simulink library "SensLib"  (R2016b)
settings: Solver=ode45  StartTime=0.0  StopTime=10.0  RelTol=1e-3  EnableMultiTasking=on
undefined symbols (not defined in the file or in its folder): AC, sens
libraries: SensLib x47, OpenFlightUtilLib x8, simulink x2
settings Model: Creator=University of Minnesota  LastModifiedBy=rega0051
settings DataIOCC: LimitDataPoints=on  SaveFormat=Array  SignalLoggingSaveFormat=ModelDataLogs
settings OptimizationCC: ExpressionDepthLimit=2147483647  LifeSpan=inf  SimCompilerOptimization=on
settings DebuggingCC: UnderspecifiedInitializationDetection=Classic  MergeDetectMultiDrivingBlocksExec=none  SolverPrmCheckMsg=warning  FcnCallInpInsideContextMsg=warning  StateNameClashWarn=warning  StrictBusMsg=Warning  SFUnexpectedBacktrackingDiag=warning  SFNoUnconditionalDefaultTransitionDiag=warning  SFExecutionAtInitializationDiag=none
settings HardwareCC: ProdBitPerPointer=32  ProdBitPerSizeT=32  ProdBitPerPtrDiffT=32  ProdLargestAtomicFloat=None  ProdIntDivRoundTo=Undefined  ProdEndianess=Unspecified  ProdWordSize=32  ProdHWDeviceType=32-bit Generic
settings ModelReferenceCC: PropagateSignalLabelsOutOfModel=off
settings GRTTargetCC: TargetLangStandard=C89/C90 (ANSI)  GeneratePreprocessorConditionals=Disable all  CombineOutputUpdateFcns=off  GRTInterface=on
settings ConfigComp: CovMetricSettings=dw  CovHtmlReporting=on  CovSaveCumulativeToWorkspaceVar=on  CovSaveSingleToWorkspaceVar=on  CovExternalEMLEnable=off

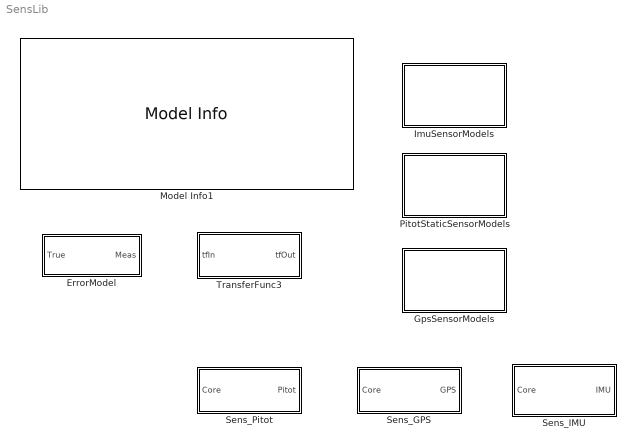
== system SensLib ==
  ErrorModel : Subsystem  mask(Sensor Error Model - Scale, Bias, Noise){enable=sens.errEnable, scf=sens.velScf, bias=sens.velBias, sigma=sens.velSigma, seed=sens.velSeed, timestep=sens.timeSample_s}
      mask prompts: enable "Enable (on/off):"; scf "Scale Factor:"; sigma "Noise Sigma:"; seed "Noise Seed:"; timestep "Time Step (s):"
      mask help:
      | Apply a scale factor, add a bias and noise to a signal.
      |
      | - Enable (on/off): 1 = error on, 0 = error off.
      | - 'Scale Factor' : Scale factor applied to original signal (applied as a matrix multiplication).
      | - 'Bias'  : Constant offset bias (vectorized).
      | - 'Sigma' : Standard deviation of noise (vectorized).
      | - 'Noise Seed'  : Random number seed (vectorized).
      | - 'Time Step (s)': Time step for the noise generation.
      mask Display: disp('bias/scf/noise')
  GpsSensorModels : Subsystem
  ImuSensorModels : Subsystem
  Model Info1 : simulink/Model-Wide Utilities/Model Info  Frame=on  DisplayStringWithTags=|  HorizontalTextAlignment=Left  LeftAlignmentValue=0.02  SourceBlockDiagram=SensLib  TagMaxNumber=20
      | MODEL INFORMATION
      | Sensors Library (%<ModelName>)
      | 
      | University of Minnesota
      | Aerospace Engineering and Mechanics
      | Copyright 2017 Regents of the University of Minnesota. All rights reserved.
      | 
      | == Update Info ==
      | Last modified by %<LastModifiedBy> on %<LastModificationDate>
  PitotStaticSensorModels : Subsystem
  Sens_GPS : Subsystem  TreatAsAtomicUnit=on  VariantControl=Variant1  mask{sens=AC.Sens.GPS}
      mask prompts: sens "GPS Parameter Structure:"
  Sens_IMU : Subsystem  TreatAsAtomicUnit=on  VariantControl=VarImu_LocTransErr  mask{sens=AC.Sens.IMU}
      mask prompts: sens "IMU Parameter Structure:"
  Sens_Pitot : Subsystem  TreatAsAtomicUnit=on  VariantControl=VarAirData_LocTransErr  mask{sens=AC.Sens.Pitot}
      mask prompts: sens "AirData Parameter Structure:"
  TransferFunc3 : Subsystem  mask(Transfer Function (3)){tf_num=sens.gyroTF_num, tf_den=sens.gyroTF_den}
      mask prompts: tf_num "Transfer Function Numerator:"; tf_den "Transfer Function Denominator:"
      mask help: Applies a Transfer Function to a vector signal of length 3. The same transfer function is applied to each signal in the vector.
      settings: AttributesFormatString=%<tf_num> / %<tf_den>

== system SensLib/ErrorModel ==
  True : Inport
  Add1 : Sum  Inputs=+++
  Band-Limited White Noise : simulink/Sources/Band-Limited White Noise  Cov=sigma  Ts=timestep  seed=seed
  Gain : Gain  Gain=scf  Multiplication=Matrix(K*u)
  Gear1 : Constant  Value=bias
  Gear2 : Constant  Value=enable
  Reshape : Reshape  OutputDimensionality=Column vector (2-D)
  Switch : Switch  Criteria=u2 > Threshold
  Meas : Outport
  wires:
  Reshape/1 -> Gain/1
  Band-Limited White Noise/1 -> Add1/3
  Gear1/1 -> Add1/2
  Add1/1 -> Switch/1
  True/1 -> Switch/3, Reshape/1
  Gain/1 -> Add1/1
  Switch/1 -> Meas/1
  Gear2/1 -> Switch/2

== system SensLib/GpsSensorModels ==
  GPS_Err : Subsystem  TreatAsAtomicUnit=on  VariantControl=Variant1
  GPS_LocErr : Subsystem  TreatAsAtomicUnit=on  VariantControl=Variant1
  GPS_LocTransErr : Subsystem  TreatAsAtomicUnit=on  VariantControl=Variant1
  GPS_Pass : Subsystem  TreatAsAtomicUnit=on  VariantControl=Variant1
  Sens_GPS : Subsystem  BlockChoice=GPS_LocErr  mask{sens=AC.Sens.GPS}
      mask prompts: sens "GPS Parameter Structure:"
      settings: TemplateBlock=self  MemberBlocks=GPS_Err,GPS_LocErr,GPS_LocTransErr,GPS_Pass
      settings: AttributesFormatString=|
      | %<BlockChoice>
      | Param Struct: %<sens>

== system SensLib/ImuSensorModels ==
  Body2IMU : Subsystem
  IMU_Err : Subsystem  TreatAsAtomicUnit=on  VariantControl=VarImu_Err
  IMU_LocErr : Subsystem  TreatAsAtomicUnit=on  VariantControl=VarImu_LocErr
  IMU_LocTransErr : Subsystem  TreatAsAtomicUnit=on  VariantControl=VarImu_LocTransErr
  IMU_Pass : Subsystem  TreatAsAtomicUnit=on  VariantControl=VarIMU_Pass
  Sens_IMU : Subsystem  BlockChoice=IMU_LocErr  mask{sens=AC.Sens.IMU}
      mask prompts: sens "Imu Param Struct:"
      settings: TemplateBlock=self  MemberBlocks=IMU_Err,IMU_LocErr,IMU_LocTransErr,IMU_Pass
      settings: AttributesFormatString=|
      | %<BlockChoice>
      | Param Struct: %<sens>

== system SensLib/PitotStaticSensorModels ==
  Body2PitotStatic : Subsystem
  Pitot_Err : Subsystem  TreatAsAtomicUnit=on  VariantControl=Variant1
  Pitot_LocErr : Subsystem  TreatAsAtomicUnit=on  VariantControl=VarAirData_LocErr
  Pitot_LocTransErr : Subsystem  TreatAsAtomicUnit=on  VariantControl=VarAirData_LocTransErr
  Pitot_Pass : Subsystem  TreatAsAtomicUnit=on  VariantControl=Variant1
  Sens_Pitot : Subsystem  BlockChoice=Pitot_Err  mask{sens=AC.Sens.Pitot}
      mask prompts: sens "Pitot Parameter Structure:"
      settings: TemplateBlock=self  MemberBlocks=Pitot_Err,Pitot_LocErr,Pitot_Pass
      settings: AttributesFormatString=|
      | %<BlockChoice>
      | Param Struct: %<sens>

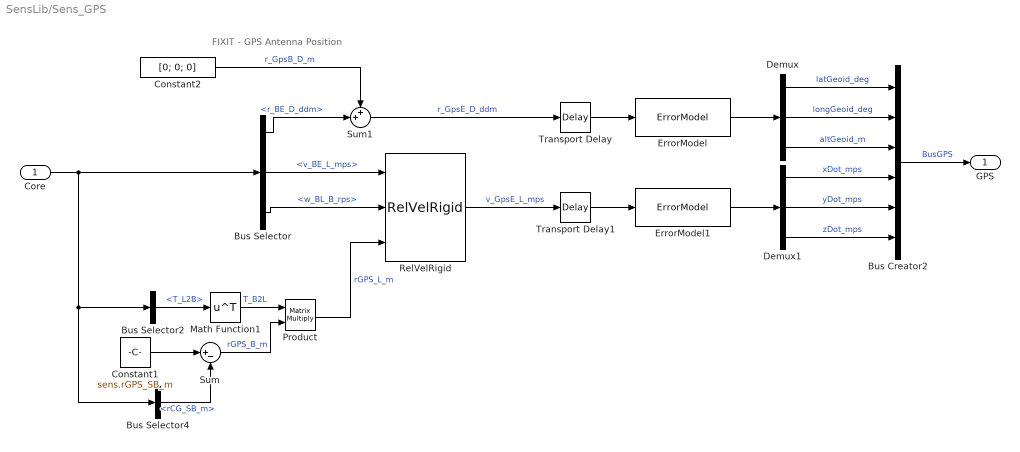
== system SensLib/Sens_GPS ==
  note: FIXIT - GPS Antenna Position
  Core : Inport
  Bus Creator2 : BusCreator  Inputs=6  OutDataTypeStr=Bus: BusGPS
      settings: InheritFromInputs=off
  Bus Selector : BusSelector  OutputSignals=BusEom.r_BE_D_ddm,BusEom.v_BE_L_mps,BusEom.w_BL_B_rps
  Bus Selector2 : BusSelector  OutputSignals=BusEom.T_L2B
  Bus Selector4 : BusSelector  OutputSignals=BusEom.rCG_SB_m
  Constant1 : Constant  Value=sens.rGPS_SB_m
      settings: AttributesFormatString=%<Value>
  Constant2 : Constant  Value=[0; 0; 0]
      settings: AttributesFormatString=%<Value>
  Demux : Demux  Outputs=3
  Demux1 : Demux  Outputs=3
  ErrorModel : SensLib/ErrorModel  enable=sens.errEnable  scf=sens.posScf  bias=sens.posBias  sigma=sens.posSigma  seed=sens.posSeed  timestep=sens.timeSample_s
  ErrorModel1 : SensLib/ErrorModel  enable=sens.errEnable  scf=sens.velScf  bias=sens.velBias  sigma=sens.velSigma  seed=sens.velSeed  timestep=sens.timeSample_s
  Math Function1 : Math  Operator=transpose  SaturateOnIntegerOverflow=on
  Product : Product  Multiplication=Matrix(*)
  RelVelRigid : OpenFlightUtilLib/Kinematics and Dynamics/RelVelRigid
  Sum : Sum  Inputs=|+-
  Sum1 : Sum  Inputs=++|
  Transport Delay : TransportDelay  DelayTime=sens.timeDelay_s  TransDelayFeedthrough=on  PadeOrder=2
      settings: AttributesFormatString=%<DelayTime>
  Transport Delay1 : TransportDelay  DelayTime=sens.timeDelay_s  TransDelayFeedthrough=on  PadeOrder=2
      settings: AttributesFormatString=%<DelayTime>
  GPS : Outport
  wires:
  Constant2/1 -> Sum1/1  "r_GpsB_D_m"
  Product/1 -> RelVelRigid/3  "rGPS_L_m"
  Math Function1/1 -> Product/1  "T_B2L"
  Bus Selector2/1 -> Math Function1/1  "<T_L2B>"
  Bus Selector/2 -> RelVelRigid/1  "<v_BE_L_mps>"
  Bus Selector4/1 -> Sum/2  "<rCG_SB_m>"
  Transport Delay1/1 -> ErrorModel1/1
  Transport Delay/1 -> ErrorModel/1
  RelVelRigid/1 -> Transport Delay1/1  "v_GpsE_L_mps"
  Sum1/1 -> Transport Delay/1  "r_GpsE_D_ddm"
  Bus Selector/1 -> Sum1/2  "<r_BE_D_ddm>"
  Sum/1 -> Product/2  "rGPS_B_m"
  Constant1/1 -> Sum/1
  ErrorModel1/1 -> Demux1/1
  ErrorModel/1 -> Demux/1
  Demux1/3 -> Bus Creator2/6  "zDot_mps"
  Demux1/2 -> Bus Creator2/5  "yDot_mps"
  Demux1/1 -> Bus Creator2/4  "xDot_mps"
  Bus Creator2/1 -> GPS/1  "BusGPS"
  Bus Selector/3 -> RelVelRigid/2  "<w_BL_B_rps>"
  Demux/3 -> Bus Creator2/3  "altGeoid_m"
  Demux/1 -> Bus Creator2/1  "latGeoid_deg"
  Demux/2 -> Bus Creator2/2  "longGeoid_deg"
  Core/1 -> Bus Selector/1, Bus Selector2/1, Bus Selector4/1

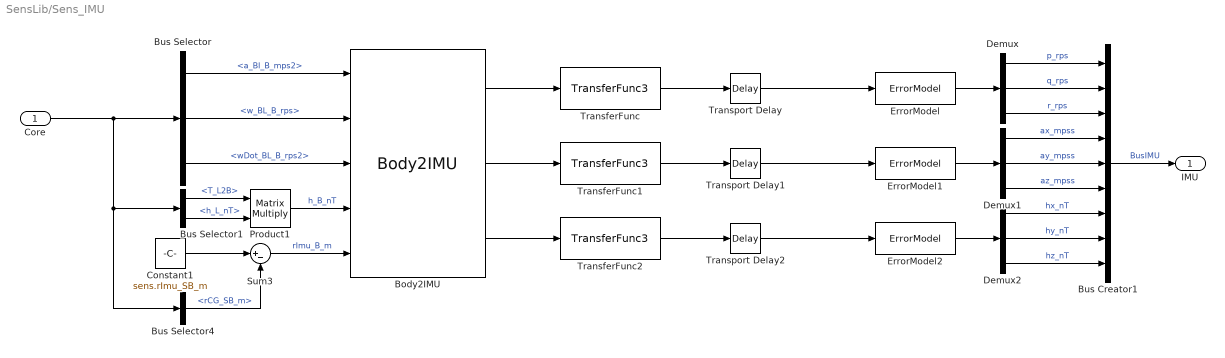
== system SensLib/Sens_IMU ==
  Core : Inport
  Body2IMU : SensLib/ImuSensorModels/Body2IMU
  Bus Creator1 : BusCreator  Inputs=9  OutDataTypeStr=Bus: BusIMU
      settings: AttributesFormatString=%<OutDataTypeStr>  InheritFromInputs=off
  Bus Selector : BusSelector  OutputSignals=BusEom.a_BI_B_mps2,BusEom.w_BL_B_rps,BusEom.wDot_BL_B_rps2
  Bus Selector1 : BusSelector  OutputSignals=BusEom.T_L2B,BusEnv.BusMag.h_L_nT
  Bus Selector4 : BusSelector  OutputSignals=BusEom.rCG_SB_m
  Constant1 : Constant  Value=sens.rImu_SB_m
      settings: AttributesFormatString=%<Value>
  Demux : Demux  Outputs=3
  Demux1 : Demux  Outputs=3
  Demux2 : Demux  Outputs=3
  ErrorModel : SensLib/ErrorModel  enable=sens.errEnable  scf=sens.gyroScf  bias=sens.gyroBias  sigma=sens.gyroSigma  seed=sens.gyroSeed  timestep=sens.timeSample_s
  ErrorModel1 : SensLib/ErrorModel  enable=sens.errEnable  scf=sens.accelScf  bias=sens.accelBias  sigma=sens.accelSigma  seed=sens.accelSeed  timestep=sens.timeSample_s
  ErrorModel2 : SensLib/ErrorModel  enable=sens.errEnable  scf=sens.magScf  bias=sens.magBias  sigma=sens.magSigma  seed=sens.magSeed  timestep=sens.timeSample_s
  Product1 : Product  Inputs=**  Multiplication=Matrix(*)  RndMeth=Zero
  Sum3 : Sum  Inputs=|+-  SaturateOnIntegerOverflow=on
  TransferFunc : SensLib/TransferFunc3  tf_num=sens.gyroTF_num  tf_den=sens.gyroTF_den
      settings: AttributesFormatString=%<tf_num> / %<tf_den>
  TransferFunc1 : SensLib/TransferFunc3  tf_num=sens.accelTF_num  tf_den=sens.accelTF_den
      settings: AttributesFormatString=%<tf_num> / %<tf_den>
  TransferFunc2 : SensLib/TransferFunc3  tf_num=sens.magTF_num  tf_den=sens.magTF_den
      settings: AttributesFormatString=%<tf_num> / %<tf_den>
  Transport Delay : TransportDelay  DelayTime=sens.timeDelay_s  TransDelayFeedthrough=on  PadeOrder=2
      settings: AttributesFormatString=%<DelayTime>
  Transport Delay1 : TransportDelay  DelayTime=sens.timeDelay_s  TransDelayFeedthrough=on  PadeOrder=2
      settings: AttributesFormatString=%<DelayTime>
  Transport Delay2 : TransportDelay  DelayTime=sens.timeDelay_s  TransDelayFeedthrough=on  PadeOrder=2
      settings: AttributesFormatString=%<DelayTime>
  IMU : Outport
  wires:
  Bus Selector1/1 -> Product1/1  "<T_L2B>"
  Bus Selector1/2 -> Product1/2  "<h_L_nT>"
  Bus Selector4/1 -> Sum3/2  "<rCG_SB_m>"
  Core/1 -> Bus Selector/1, Bus Selector1/1, Bus Selector4/1
  Bus Creator1/1 -> IMU/1  "BusIMU"
  Demux/1 -> Bus Creator1/1  "p_rps"
  Demux1/1 -> Bus Creator1/4  "ax_mpss"
  Demux1/2 -> Bus Creator1/5  "ay_mpss"
  Demux1/3 -> Bus Creator1/6  "az_mpss"
  Demux/2 -> Bus Creator1/2  "q_rps"
  Demux/3 -> Bus Creator1/3  "r_rps"
  Demux2/1 -> Bus Creator1/7  "hx_nT"
  Demux2/2 -> Bus Creator1/8  "hy_nT"
  Demux2/3 -> Bus Creator1/9  "hz_nT"
  ErrorModel/1 -> Demux/1
  ErrorModel1/1 -> Demux1/1
  ErrorModel2/1 -> Demux2/1
  Body2IMU/1 -> TransferFunc/1
  TransferFunc/1 -> Transport Delay/1
  Body2IMU/2 -> TransferFunc1/1
  Body2IMU/3 -> TransferFunc2/1
  TransferFunc1/1 -> Transport Delay1/1
  TransferFunc2/1 -> Transport Delay2/1
  Transport Delay/1 -> ErrorModel/1
  Transport Delay1/1 -> ErrorModel1/1
  Transport Delay2/1 -> ErrorModel2/1
  Product1/1 -> Body2IMU/4  "h_B_nT"
  Bus Selector/1 -> Body2IMU/1  "<a_BI_B_mps2>"
  Bus Selector/2 -> Body2IMU/2  "<w_BL_B_rps>"
  Bus Selector/3 -> Body2IMU/3  "<wDot_BL_B_rps2>"
  Constant1/1 -> Sum3/1
  Sum3/1 -> Body2IMU/5  "rImu_B_m"

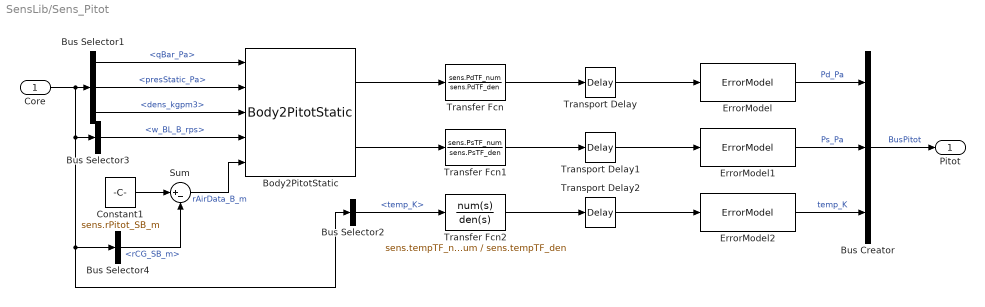
== system SensLib/Sens_Pitot ==
  Core : Inport
  Body2PitotStatic : SensLib/PitotStaticSensorModels/Body2PitotStatic
  Bus Creator : BusCreator  Inputs=3  OutDataTypeStr=Bus: BusPitot
      settings: AttributesFormatString=%<OutDataTypeStr>  InheritFromInputs=off
  Bus Selector1 : BusSelector  OutputSignals=BusAux.BusFlow.qBar_Pa,BusEnv.BusAtmos.presStatic_Pa,BusEnv.BusAtmos.dens_kgpm3
  Bus Selector2 : BusSelector  OutputSignals=BusEnv.BusAtmos.temp_K
  Bus Selector3 : BusSelector  OutputSignals=BusEom.w_BL_B_rps
  Bus Selector4 : BusSelector  OutputSignals=BusEom.rCG_SB_m
  Constant1 : Constant  Value=sens.rPitot_SB_m
      settings: AttributesFormatString=%<Value>
  ErrorModel : SensLib/ErrorModel  enable=sens.errEnable  scf=sens.PdScf  bias=sens.PdBias  sigma=sens.PdSigma  seed=sens.PdSeed  timestep=sens.timeSample_s
  ErrorModel1 : SensLib/ErrorModel  enable=sens.errEnable  scf=sens.PsScf  bias=sens.PsBias  sigma=sens.PsSigma  seed=sens.PsSeed  timestep=sens.timeSample_s
  ErrorModel2 : SensLib/ErrorModel  enable=sens.errEnable  scf=sens.tempScf  bias=sens.tempBias  sigma=sens.tempSigma  seed=sens.tempSeed  timestep=sens.timeSample_s
  Sum : Sum  Inputs=|+-
  Transfer Fcn : TransferFcn  Numerator=sens.PdTF_num  Denominator=sens.PdTF_den
      settings: AttributesFormatString=|
      | %<Numerator>
      | %<Denominator>
  Transfer Fcn1 : TransferFcn  Numerator=sens.PsTF_num  Denominator=sens.PsTF_den
      settings: AttributesFormatString=|
      | %<Numerator>
      | %<Denominator>
  Transfer Fcn2 : TransferFcn  Numerator=sens.tempTF_num  Denominator=sens.tempTF_den
      settings: AttributesFormatString=|
      | %<Numerator>
      | %<Denominator>
  Transport Delay : TransportDelay  DelayTime=sens.PdTimeDelay_s  TransDelayFeedthrough=on  PadeOrder=2
      settings: AttributesFormatString=%<DelayTime>
  Transport Delay1 : TransportDelay  DelayTime=sens.PdTimeDelay_s  TransDelayFeedthrough=on  PadeOrder=2
      settings: AttributesFormatString=%<DelayTime>
  Transport Delay2 : TransportDelay  DelayTime=sens.tempTimeDelay_s  TransDelayFeedthrough=on  PadeOrder=2
      settings: AttributesFormatString=%<DelayTime>
  Pitot : Outport
  wires:
  Bus Creator/1 -> Pitot/1  "BusPitot"
  ErrorModel/1 -> Bus Creator/1  "Pd_Pa"
  ErrorModel1/1 -> Bus Creator/2  "Ps_Pa"
  ErrorModel2/1 -> Bus Creator/3  "temp_K"
  Body2PitotStatic/1 -> Transfer Fcn/1
  Body2PitotStatic/2 -> Transfer Fcn1/1
  Transfer Fcn/1 -> Transport Delay/1
  Transfer Fcn1/1 -> Transport Delay1/1
  Transfer Fcn2/1 -> Transport Delay2/1
  Transport Delay/1 -> ErrorModel/1
  Transport Delay1/1 -> ErrorModel1/1
  Transport Delay2/1 -> ErrorModel2/1
  Bus Selector3/1 -> Body2PitotStatic/4  "<w_BL_B_rps>"
  Bus Selector1/3 -> Body2PitotStatic/3  "<dens_kgpm3>"
  Core/1 -> Bus Selector3/1, Bus Selector4/1, Bus Selector2/1, Bus Selector1/1
  Bus Selector1/1 -> Body2PitotStatic/1  "<qBar_Pa>"
  Bus Selector1/2 -> Body2PitotStatic/2  "<presStatic_Pa>"
  Bus Selector2/1 -> Transfer Fcn2/1  "<temp_K>"
  Bus Selector4/1 -> Sum/2  "<rCG_SB_m>"
  Constant1/1 -> Sum/1
  Sum/1 -> Body2PitotStatic/5  "rAirData_B_m"

== system SensLib/TransferFunc3 ==
  tfIn : Inport
  Demux : Demux  Outputs=3
  Mux : Mux  Inputs=3
  Transfer Fcn : TransferFcn  Numerator=tf_num  Denominator=tf_den
  Transfer Fcn1 : TransferFcn  Numerator=tf_num  Denominator=tf_den
  Transfer Fcn2 : TransferFcn  Numerator=tf_num  Denominator=tf_den
  tfOut : Outport
  wires:
  tfIn/1 -> Demux/1
  Mux/1 -> tfOut/1
  Demux/1 -> Transfer Fcn/1
  Demux/2 -> Transfer Fcn1/1
  Demux/3 -> Transfer Fcn2/1
  Transfer Fcn/1 -> Mux/1
  Transfer Fcn1/1 -> Mux/2
  Transfer Fcn2/1 -> Mux/3

== system SensLib/GpsSensorModels/GPS_Err ==
  Core : Inport
  Bus Creator2 : BusCreator  Inputs=6  OutDataTypeStr=Bus: BusGPS
      settings: AttributesFormatString=%<OutDataTypeStr>  InheritFromInputs=off
  Bus Selector : BusSelector  OutputSignals=AuxVar.Nav.GeodeticLatitude_deg,AuxVar.Nav.GeodeticLongitude_deg,AuxVar.Nav.Altitude_m,AuxVar.V_e.Xdot_mps,AuxVar.V_e.Ydot_mps,AuxVar.V_e.Zdot_mps
  Demux : Demux  Outputs=3
  Demux1 : Demux  Outputs=3
  ErrorModel : SensLib/ErrorModel  enable=sens.errEnable  scf=sens.posScf  bias=sens.posBias  sigma=sens.posSigma  seed=sens.posSeed  timestep=sens.timeSample_s
  ErrorModel1 : SensLib/ErrorModel  enable=sens.errEnable  scf=sens.velScf  bias=sens.velBias  sigma=sens.velSigma  seed=sens.velSeed  timestep=sens.timeSample_s
  Mux : Mux  Inputs=3
  Mux1 : Mux  Inputs=3
  GPS : Outport
  wires:
  Core/1 -> Bus Selector/1
  Demux/2 -> Bus Creator2/2  "longGeoid_deg"
  Demux/1 -> Bus Creator2/1  "latGeoid_deg"
  Demux/3 -> Bus Creator2/3  "altGeoid_m"
  Bus Selector/1 -> Mux/1  "<GeodeticLatitude_deg>"
  Bus Selector/2 -> Mux/2  "<GeodeticLongitude_deg>"
  Bus Selector/3 -> Mux/3  "<Altitude_m>"
  Bus Selector/6 -> Mux1/3  "<Zdot_mps>"
  Bus Selector/5 -> Mux1/2  "<Ydot_mps>"
  Bus Selector/4 -> Mux1/1  "<Xdot_mps>"
  Bus Creator2/1 -> GPS/1  "BusGPS"
  Mux/1 -> ErrorModel/1
  Demux1/1 -> Bus Creator2/4  "xDot_mps"
  Demux1/2 -> Bus Creator2/5  "yDot_mps"
  Demux1/3 -> Bus Creator2/6  "zDot_mps"
  ErrorModel/1 -> Demux/1
  Mux1/1 -> ErrorModel1/1
  ErrorModel1/1 -> Demux1/1

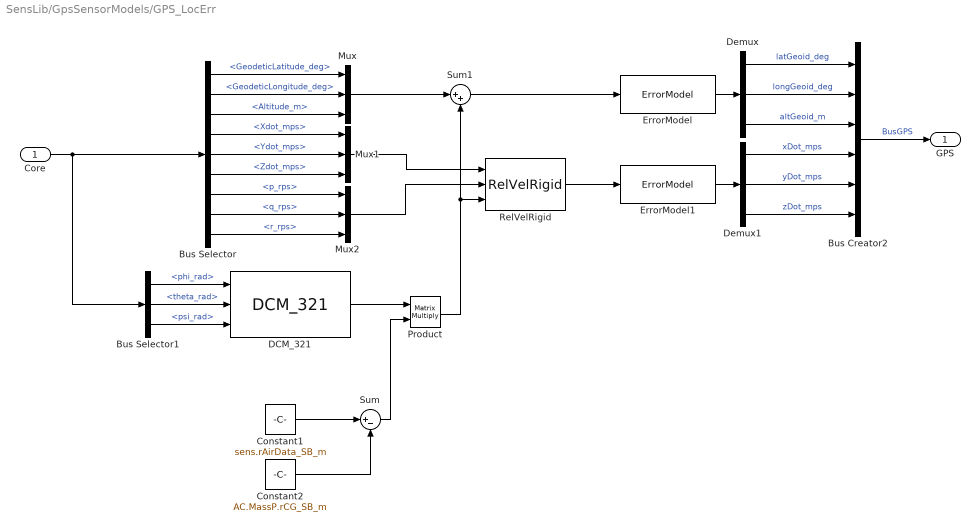
== system SensLib/GpsSensorModels/GPS_LocErr ==
  Core : Inport
  Bus Creator2 : BusCreator  Inputs=6  OutDataTypeStr=Bus: BusGPS
      settings: AttributesFormatString=%<OutDataTypeStr>  InheritFromInputs=off
  Bus Selector : BusSelector  OutputSignals=AuxVar.Nav.GeodeticLatitude_deg,AuxVar.Nav.GeodeticLongitude_deg,AuxVar.Nav.Altitude_m,AuxVar.V_e.Xdot_mps,AuxVar.V_e.Ydot_mps,AuxVar.V_e.Zdot_mps,RigidStates.AngVel.p_rps,RigidStates.AngVel.q_rps,RigidStates.AngVel.r_rps
  Bus Selector1 : BusSelector  OutputSignals=RigidStates.Euler.phi_rad,RigidStates.Euler.theta_rad,RigidStates.Euler.psi_rad
  Constant1 : Constant  Value=sens.rAirData_SB_m
      settings: AttributesFormatString=%<Value>
  Constant2 : Constant  Value=AC.MassP.rCG_SB_m
      settings: AttributesFormatString=%<Value>
  DCM_321 : OpenFlightUtilLib/Transformations/DCM_321
  Demux : Demux  Outputs=3
  Demux1 : Demux  Outputs=3
  ErrorModel : SensLib/ErrorModel  enable=sens.errEnable  scf=sens.posScf  bias=sens.posBias  sigma=sens.posSigma  seed=sens.posSeed  timestep=sens.timeSample_s
  ErrorModel1 : SensLib/ErrorModel  enable=sens.errEnable  scf=sens.velScf  bias=sens.velBias  sigma=sens.velSigma  seed=sens.velSeed  timestep=sens.timeSample_s
  Mux : Mux  Inputs=3
  Mux1 : Mux  Inputs=3
  Mux2 : Mux  Inputs=3
  Product : Product  Multiplication=Matrix(*)
  RelVelRigid : OpenFlightUtilLib/Kinematics and Dynamics/RelVelRigid
  Sum : Sum  Inputs=|+-
  Sum1 : Sum  Inputs=|++
  GPS : Outport
  wires:
  Core/1 -> Bus Selector1/1, Bus Selector/1
  Demux/2 -> Bus Creator2/2  "longGeoid_deg"
  Demux/1 -> Bus Creator2/1  "latGeoid_deg"
  Demux/3 -> Bus Creator2/3  "altGeoid_m"
  Bus Selector/1 -> Mux/1  "<GeodeticLatitude_deg>"
  Bus Selector/2 -> Mux/2  "<GeodeticLongitude_deg>"
  Bus Selector/3 -> Mux/3  "<Altitude_m>"
  Bus Selector/6 -> Mux1/3  "<Zdot_mps>"
  Bus Selector/5 -> Mux1/2  "<Ydot_mps>"
  Bus Selector/4 -> Mux1/1  "<Xdot_mps>"
  Bus Creator2/1 -> GPS/1  "BusGPS"
  Demux1/1 -> Bus Creator2/4  "xDot_mps"
  Demux1/2 -> Bus Creator2/5  "yDot_mps"
  Demux1/3 -> Bus Creator2/6  "zDot_mps"
  ErrorModel/1 -> Demux/1
  ErrorModel1/1 -> Demux1/1
  Constant1/1 -> Sum/1
  Constant2/1 -> Sum/2
  Sum/1 -> Product/2
  DCM_321/1 -> Product/1
  Product/1 -> Sum1/2, RelVelRigid/3
  Mux/1 -> Sum1/1
  Sum1/1 -> ErrorModel/1
  RelVelRigid/1 -> ErrorModel1/1
  Mux1/1 -> RelVelRigid/1
  Bus Selector1/1 -> DCM_321/1  "<phi_rad>"
  Bus Selector1/2 -> DCM_321/2  "<theta_rad>"
  Bus Selector1/3 -> DCM_321/3  "<psi_rad>"
  Mux2/1 -> RelVelRigid/2
  Bus Selector/8 -> Mux2/2  "<q_rps>"
  Bus Selector/7 -> Mux2/1  "<p_rps>"
  Bus Selector/9 -> Mux2/3  "<r_rps>"

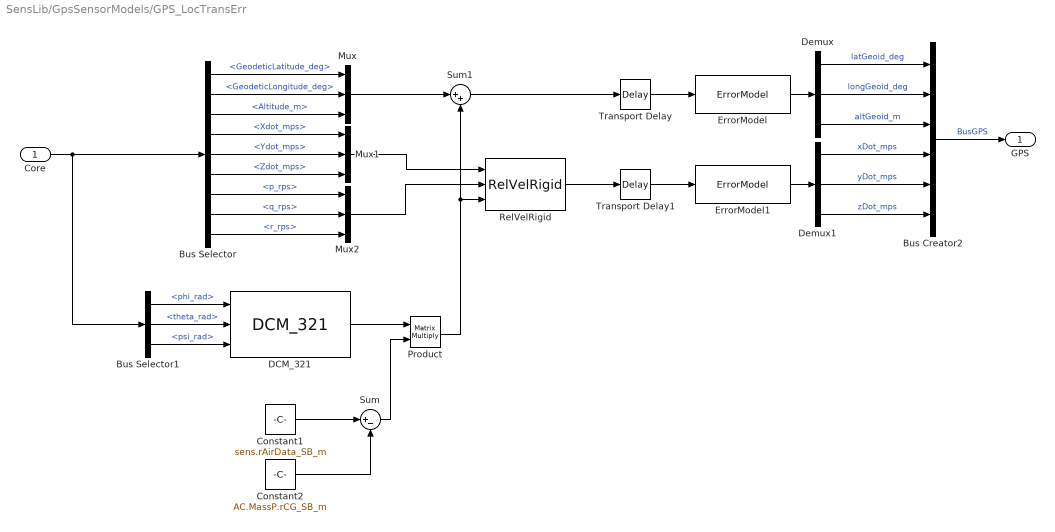
== system SensLib/GpsSensorModels/GPS_LocTransErr ==
  Core : Inport
  Bus Creator2 : BusCreator  Inputs=6  OutDataTypeStr=Bus: BusGPS
      settings: AttributesFormatString=%<OutDataTypeStr>  InheritFromInputs=off
  Bus Selector : BusSelector  OutputSignals=AuxVar.Nav.GeodeticLatitude_deg,AuxVar.Nav.GeodeticLongitude_deg,AuxVar.Nav.Altitude_m,AuxVar.V_e.Xdot_mps,AuxVar.V_e.Ydot_mps,AuxVar.V_e.Zdot_mps,RigidStates.AngVel.p_rps,RigidStates.AngVel.q_rps,RigidStates.AngVel.r_rps
  Bus Selector1 : BusSelector  OutputSignals=RigidStates.Euler.phi_rad,RigidStates.Euler.theta_rad,RigidStates.Euler.psi_rad
  Constant1 : Constant  Value=sens.rAirData_SB_m
      settings: AttributesFormatString=%<Value>
  Constant2 : Constant  Value=AC.MassP.rCG_SB_m
      settings: AttributesFormatString=%<Value>
  DCM_321 : OpenFlightUtilLib/Transformations/DCM_321
  Demux : Demux  Outputs=3
  Demux1 : Demux  Outputs=3
  ErrorModel : SensLib/ErrorModel  enable=sens.errEnable  scf=sens.posScf  bias=sens.posBias  sigma=sens.posSigma  seed=sens.posSeed  timestep=sens.timeSample_s
  ErrorModel1 : SensLib/ErrorModel  enable=sens.errEnable  scf=sens.velScf  bias=sens.velBias  sigma=sens.velSigma  seed=sens.velSeed  timestep=sens.timeSample_s
  Mux : Mux  Inputs=3
  Mux1 : Mux  Inputs=3
  Mux2 : Mux  Inputs=3
  Product : Product  Multiplication=Matrix(*)
  RelVelRigid : OpenFlightUtilLib/Kinematics and Dynamics/RelVelRigid
  Sum : Sum  Inputs=|+-
  Sum1 : Sum  Inputs=|++
  Transport Delay : TransportDelay  DelayTime=sens.timeDelay_s  TransDelayFeedthrough=on  PadeOrder=2
      settings: AttributesFormatString=%<DelayTime>
  Transport Delay1 : TransportDelay  DelayTime=sens.timeDelay_s  TransDelayFeedthrough=on  PadeOrder=2
      settings: AttributesFormatString=%<DelayTime>
  GPS : Outport
  wires:
  Transport Delay1/1 -> ErrorModel1/1
  Transport Delay/1 -> ErrorModel/1
  Bus Selector/9 -> Mux2/3  "<r_rps>"
  Bus Selector/7 -> Mux2/1  "<p_rps>"
  Bus Selector/8 -> Mux2/2  "<q_rps>"
  Mux2/1 -> RelVelRigid/2
  Bus Selector1/3 -> DCM_321/3  "<psi_rad>"
  Bus Selector1/2 -> DCM_321/2  "<theta_rad>"
  Bus Selector1/1 -> DCM_321/1  "<phi_rad>"
  Mux1/1 -> RelVelRigid/1
  RelVelRigid/1 -> Transport Delay1/1
  Sum1/1 -> Transport Delay/1
  Mux/1 -> Sum1/1
  Product/1 -> RelVelRigid/3, Sum1/2
  DCM_321/1 -> Product/1
  Sum/1 -> Product/2
  Constant2/1 -> Sum/2
  Constant1/1 -> Sum/1
  ErrorModel1/1 -> Demux1/1
  ErrorModel/1 -> Demux/1
  Demux1/3 -> Bus Creator2/6  "zDot_mps"
  Demux1/2 -> Bus Creator2/5  "yDot_mps"
  Demux1/1 -> Bus Creator2/4  "xDot_mps"
  Bus Creator2/1 -> GPS/1  "BusGPS"
  Bus Selector/4 -> Mux1/1  "<Xdot_mps>"
  Bus Selector/5 -> Mux1/2  "<Ydot_mps>"
  Bus Selector/6 -> Mux1/3  "<Zdot_mps>"
  Bus Selector/3 -> Mux/3  "<Altitude_m>"
  Bus Selector/2 -> Mux/2  "<GeodeticLongitude_deg>"
  Bus Selector/1 -> Mux/1  "<GeodeticLatitude_deg>"
  Demux/3 -> Bus Creator2/3  "altGeoid_m"
  Demux/1 -> Bus Creator2/1  "latGeoid_deg"
  Demux/2 -> Bus Creator2/2  "longGeoid_deg"
  Core/1 -> Bus Selector/1, Bus Selector1/1

== system SensLib/GpsSensorModels/GPS_Pass ==
  Core : Inport
  Bus Creator2 : BusCreator  Inputs=6  OutDataTypeStr=Bus: BusGPS
      settings: AttributesFormatString=%<OutDataTypeStr>
  Bus Selector : BusSelector  OutputSignals=AuxVar.Nav.GeodeticLatitude_deg,AuxVar.Nav.GeodeticLongitude_deg,AuxVar.Nav.Altitude_m,AuxVar.V_e.Xdot_mps,AuxVar.V_e.Ydot_mps,AuxVar.V_e.Zdot_mps
  GPS : Outport
  wires:
  Core/1 -> Bus Selector/1
  Bus Selector/1 -> Bus Creator2/1  "<GeodeticLatitude_deg>"
  Bus Selector/3 -> Bus Creator2/3  "<Altitude_m>"
  Bus Selector/2 -> Bus Creator2/2  "<GeodeticLongitude_deg>"
  Bus Selector/6 -> Bus Creator2/6  "<Zdot_mps>"
  Bus Selector/4 -> Bus Creator2/4  "<Xdot_mps>"
  Bus Creator2/1 -> GPS/1  "BusGPS"
  Bus Selector/5 -> Bus Creator2/5  "<Ydot_mps>"

== system SensLib/GpsSensorModels/Sens_GPS ==
  Core : Inport
  GPS_LocErr : SensLib/GpsSensorModels/GPS_LocErr  VariantControl=Variant1
  GPS : Outport
  wires:
  Core/1 -> GPS_LocErr/1
  GPS_LocErr/1 -> GPS/1

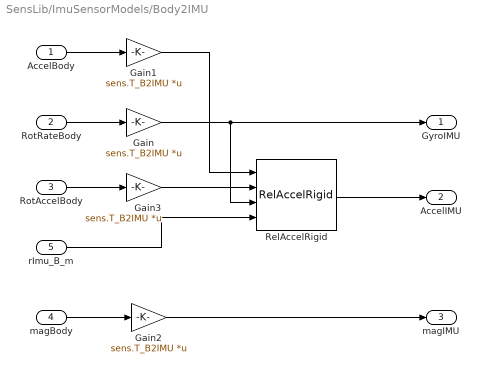
== system SensLib/ImuSensorModels/Body2IMU ==
  AccelBody : Inport
  RotRateBody : Inport  Port=2
  RotAccelBody : Inport  Port=3
  magBody : Inport  Port=4
  rImu_B_m : Inport  Port=5
  Gain{,1..3} (4 alike) : Gain  Gain=sens.T_B2IMU  Multiplication=Matrix(K*u)
      settings: AttributesFormatString=%<Gain>
  RelAccelRigid : OpenFlightUtilLib/Kinematics and Dynamics/RelAccelRigid
  GyroIMU : Outport
  AccelIMU : Outport  Port=2
  magIMU : Outport  Port=3
  wires:
  RotRateBody/1 -> Gain/1
  AccelBody/1 -> Gain1/1
  rImu_B_m/1 -> RelAccelRigid/4
  RelAccelRigid/1 -> AccelIMU/1
  Gain2/1 -> magIMU/1
  Gain1/1 -> RelAccelRigid/1
  Gain/1 -> GyroIMU/1, RelAccelRigid/3
  RotAccelBody/1 -> Gain3/1
  Gain3/1 -> RelAccelRigid/2
  magBody/1 -> Gain2/1

== system SensLib/ImuSensorModels/IMU_Err ==
  Core : Inport
  Bus Creator1 : BusCreator  Inputs=9  OutDataTypeStr=Bus: BusIMU
      settings: AttributesFormatString=%<OutDataTypeStr>  InheritFromInputs=off
  Bus Selector : BusSelector  OutputSignals=RigidStates.AngVel.p_rps,RigidStates.AngVel.q_rps,RigidStates.AngVel.r_rps,RigidStates.Accels.Ax_mpss,RigidStates.Accels.Ay_mpss,RigidStates.Accels.Az_mpss,EnvData.MageneticField_nT
  Demux : Demux  Outputs=3
  Demux1 : Demux  Outputs=3
  Demux2 : Demux  Outputs=3
  ErrorModel : SensLib/ErrorModel  enable=sens.errEnable  scf=sens.gyroScf  bias=sens.gyroBias  sigma=sens.gyroSigma  seed=sens.gyroSeed  timestep=sens.timeSample_s
  ErrorModel1 : SensLib/ErrorModel  enable=sens.errEnable  scf=sens.accelScf  bias=sens.accelBias  sigma=sens.accelSigma  seed=sens.accelSeed  timestep=sens.timeSample_s
  ErrorModel2 : SensLib/ErrorModel  enable=sens.errEnable  scf=sens.magScf  bias=sens.magBias  sigma=sens.magSigma  seed=sens.magSeed  timestep=sens.timeSample_s
  Mux : Mux  Inputs=3
  Mux1 : Mux  Inputs=3
  IMU : Outport
  wires:
  Demux2/3 -> Bus Creator1/9  "hz_nT"
  Demux2/2 -> Bus Creator1/8  "hy_nT"
  Demux2/1 -> Bus Creator1/7  "hx_nT"
  ErrorModel2/1 -> Demux2/1
  Bus Selector/7 -> ErrorModel2/1  "<MageneticField_nT>"
  ErrorModel1/1 -> Demux1/1
  Mux1/1 -> ErrorModel1/1
  Demux/3 -> Bus Creator1/3  "r_rps"
  Demux/2 -> Bus Creator1/2  "q_rps"
  Mux/1 -> ErrorModel/1
  ErrorModel/1 -> Demux/1
  Demux1/3 -> Bus Creator1/6  "az_mpss"
  Demux1/2 -> Bus Creator1/5  "ay_mpss"
  Demux1/1 -> Bus Creator1/4  "ax_mpss"
  Demux/1 -> Bus Creator1/1  "p_rps"
  Bus Creator1/1 -> IMU/1  "BusIMU"
  Bus Selector/6 -> Mux1/3  "<Az_mpss>"
  Bus Selector/5 -> Mux1/2  "<Ay_mpss>"
  Bus Selector/4 -> Mux1/1  "<Ax_mpss>"
  Bus Selector/3 -> Mux/3  "<r_rps>"
  Bus Selector/2 -> Mux/2  "<q_rps>"
  Bus Selector/1 -> Mux/1  "<p_rps>"
  Core/1 -> Bus Selector/1

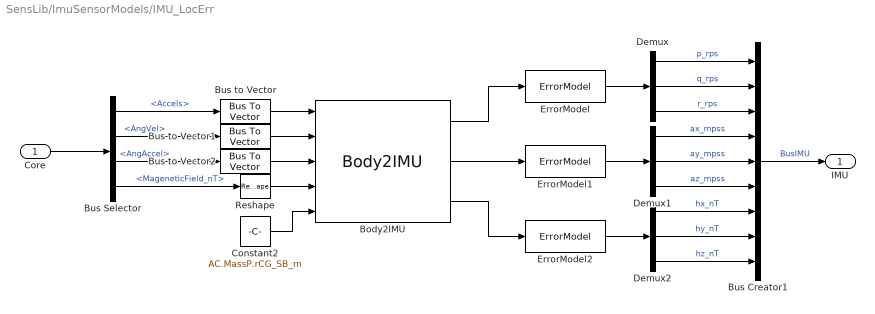
== system SensLib/ImuSensorModels/IMU_LocErr ==
  Core : Inport
  Body2IMU : SensLib/ImuSensorModels/Body2IMU
  Bus Creator1 : BusCreator  Inputs=9  OutDataTypeStr=Bus: BusIMU
      settings: AttributesFormatString=%<OutDataTypeStr>  InheritFromInputs=off
  Bus Selector : BusSelector  OutputSignals=RigidStates.Accels,RigidStates.AngVel,RigidStates.AngAccel,EnvData.MageneticField_nT
  Bus to Vector : BusToVector
  Bus to Vector1 : BusToVector
  Bus to Vector2 : BusToVector
  Constant2 : Constant  Value=AC.MassP.rCG_SB_m
      settings: AttributesFormatString=%<Value>
  Demux : Demux  Outputs=3
  Demux1 : Demux  Outputs=3
  Demux2 : Demux  Outputs=3
  ErrorModel : SensLib/ErrorModel  enable=sens.errEnable  scf=sens.gyroScf  bias=sens.gyroBias  sigma=sens.gyroSigma  seed=sens.gyroSeed  timestep=sens.timeSample_s
  ErrorModel1 : SensLib/ErrorModel  enable=sens.errEnable  scf=sens.accelScf  bias=sens.accelBias  sigma=sens.accelSigma  seed=sens.accelSeed  timestep=sens.timeSample_s
  ErrorModel2 : SensLib/ErrorModel  enable=sens.errEnable  scf=sens.magScf  bias=sens.magBias  sigma=sens.magSigma  seed=sens.magSeed  timestep=sens.timeSample_s
  Reshape : Reshape  OutputDimensionality=Column vector (2-D)
  IMU : Outport
  wires:
  Core/1 -> Bus Selector/1
  Bus Creator1/1 -> IMU/1  "BusIMU"
  Demux/1 -> Bus Creator1/1  "p_rps"
  Demux1/1 -> Bus Creator1/4  "ax_mpss"
  Demux1/2 -> Bus Creator1/5  "ay_mpss"
  Demux1/3 -> Bus Creator1/6  "az_mpss"
  Demux/2 -> Bus Creator1/2  "q_rps"
  Demux/3 -> Bus Creator1/3  "r_rps"
  Demux2/1 -> Bus Creator1/7  "hx_nT"
  Demux2/2 -> Bus Creator1/8  "hy_nT"
  Demux2/3 -> Bus Creator1/9  "hz_nT"
  ErrorModel/1 -> Demux/1
  ErrorModel1/1 -> Demux1/1
  ErrorModel2/1 -> Demux2/1
  Bus Selector/4 -> Reshape/1  "<MageneticField_nT>"
  Body2IMU/1 -> ErrorModel/1
  Body2IMU/2 -> ErrorModel1/1
  Body2IMU/3 -> ErrorModel2/1
  Reshape/1 -> Body2IMU/4
  Bus to Vector/1 -> Body2IMU/1
  Bus to Vector1/1 -> Body2IMU/2
  Bus to Vector2/1 -> Body2IMU/3
  Bus Selector/1 -> Bus to Vector/1  "<Accels>"
  Bus Selector/2 -> Bus to Vector1/1  "<AngVel>"
  Bus Selector/3 -> Bus to Vector2/1  "<AngAccel>"
  Constant2/1 -> Body2IMU/5

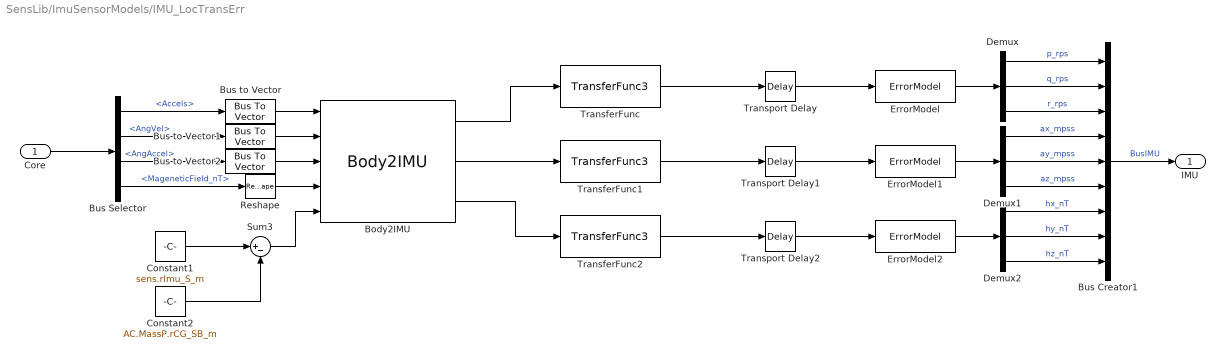
== system SensLib/ImuSensorModels/IMU_LocTransErr ==
  Core : Inport
  Body2IMU : SensLib/ImuSensorModels/Body2IMU
  Bus Creator1 : BusCreator  Inputs=9  OutDataTypeStr=Bus: BusIMU
      settings: AttributesFormatString=%<OutDataTypeStr>  InheritFromInputs=off
  Bus Selector : BusSelector  OutputSignals=RigidStates.Accels,RigidStates.AngVel,RigidStates.AngAccel,EnvData.MageneticField_nT
  Bus to Vector : BusToVector
  Bus to Vector1 : BusToVector
  Bus to Vector2 : BusToVector
  Constant1 : Constant  Value=sens.rImu_S_m
      settings: AttributesFormatString=%<Value>
  Constant2 : Constant  Value=AC.MassP.rCG_SB_m
      settings: AttributesFormatString=%<Value>
  Demux : Demux  Outputs=3
  Demux1 : Demux  Outputs=3
  Demux2 : Demux  Outputs=3
  ErrorModel : SensLib/ErrorModel  enable=sens.errEnable  scf=sens.gyroScf  bias=sens.gyroBias  sigma=sens.gyroSigma  seed=sens.gyroSeed  timestep=sens.timeSample_s
  ErrorModel1 : SensLib/ErrorModel  enable=sens.errEnable  scf=sens.accelScf  bias=sens.accelBias  sigma=sens.accelSigma  seed=sens.accelSeed  timestep=sens.timeSample_s
  ErrorModel2 : SensLib/ErrorModel  enable=sens.errEnable  scf=sens.magScf  bias=sens.magBias  sigma=sens.magSigma  seed=sens.magSeed  timestep=sens.timeSample_s
  Reshape : Reshape  OutputDimensionality=Column vector (2-D)
  Sum3 : Sum  Inputs=|+-  SaturateOnIntegerOverflow=on
  TransferFunc : SensLib/TransferFunc3  tf_num=sens.gyroTF_num  tf_den=sens.gyroTF_den
      settings: AttributesFormatString=%<tf_num> / %<tf_den>
  TransferFunc1 : SensLib/TransferFunc3  tf_num=sens.accelTF_num  tf_den=sens.accelTF_den
      settings: AttributesFormatString=%<tf_num> / %<tf_den>
  TransferFunc2 : SensLib/TransferFunc3  tf_num=sens.magTF_num  tf_den=sens.magTF_den
      settings: AttributesFormatString=%<tf_num> / %<tf_den>
  Transport Delay : TransportDelay  DelayTime=sens.timeDelay_s  TransDelayFeedthrough=on  PadeOrder=2
      settings: AttributesFormatString=%<DelayTime>
  Transport Delay1 : TransportDelay  DelayTime=sens.timeDelay_s  TransDelayFeedthrough=on  PadeOrder=2
      settings: AttributesFormatString=%<DelayTime>
  Transport Delay2 : TransportDelay  DelayTime=sens.timeDelay_s  TransDelayFeedthrough=on  PadeOrder=2
      settings: AttributesFormatString=%<DelayTime>
  IMU : Outport
  wires:
  Bus Creator1/1 -> IMU/1  "BusIMU"
  Demux/1 -> Bus Creator1/1  "p_rps"
  Demux1/1 -> Bus Creator1/4  "ax_mpss"
  Demux1/2 -> Bus Creator1/5  "ay_mpss"
  Demux1/3 -> Bus Creator1/6  "az_mpss"
  Demux/2 -> Bus Creator1/2  "q_rps"
  Demux/3 -> Bus Creator1/3  "r_rps"
  Demux2/1 -> Bus Creator1/7  "hx_nT"
  Demux2/2 -> Bus Creator1/8  "hy_nT"
  Demux2/3 -> Bus Creator1/9  "hz_nT"
  ErrorModel/1 -> Demux/1
  ErrorModel1/1 -> Demux1/1
  ErrorModel2/1 -> Demux2/1
  Body2IMU/1 -> TransferFunc/1
  TransferFunc/1 -> Transport Delay/1
  Body2IMU/2 -> TransferFunc1/1
  Body2IMU/3 -> TransferFunc2/1
  TransferFunc1/1 -> Transport Delay1/1
  TransferFunc2/1 -> Transport Delay2/1
  Transport Delay/1 -> ErrorModel/1
  Transport Delay1/1 -> ErrorModel1/1
  Transport Delay2/1 -> ErrorModel2/1
  Core/1 -> Bus Selector/1
  Bus Selector/4 -> Reshape/1  "<MageneticField_nT>"
  Reshape/1 -> Body2IMU/4
  Bus to Vector/1 -> Body2IMU/1
  Bus to Vector1/1 -> Body2IMU/2
  Bus to Vector2/1 -> Body2IMU/3
  Bus Selector/1 -> Bus to Vector/1  "<Accels>"
  Bus Selector/2 -> Bus to Vector1/1  "<AngVel>"
  Bus Selector/3 -> Bus to Vector2/1  "<AngAccel>"
  Constant2/1 -> Sum3/2
  Constant1/1 -> Sum3/1
  Sum3/1 -> Body2IMU/5

== system SensLib/ImuSensorModels/IMU_Pass ==
  note: IMU Passthrough Model
  Core : Inport
  Bus Creator1 : BusCreator  Inputs=9  OutDataTypeStr=Bus: BusIMU
      settings: AttributesFormatString=%<OutDataTypeStr>  InheritFromInputs=off
  Bus Selector : BusSelector  OutputSignals=RigidStates.AngVel.p_rps,RigidStates.AngVel.q_rps,RigidStates.AngVel.r_rps,RigidStates.Accels.Ax_mpss,RigidStates.Accels.Ay_mpss,RigidStates.Accels.Az_mpss,EnvData.MageneticField_nT
  Demux3 : Demux  Outputs=3
  IMU : Outport
  wires:
  Demux3/3 -> Bus Creator1/9  "hZ_nT"
  Demux3/2 -> Bus Creator1/8  "hY_nT"
  Demux3/1 -> Bus Creator1/7  "hX_nT"
  Bus Selector/7 -> Demux3/1  "<MageneticField_nT>"
  Bus Selector/5 -> Bus Creator1/5  "<Ay_mpss>"
  Bus Creator1/1 -> IMU/1  "BusIMU"
  Bus Selector/4 -> Bus Creator1/4  "<Ax_mpss>"
  Bus Selector/3 -> Bus Creator1/3  "<r_rps>"
  Bus Selector/2 -> Bus Creator1/2  "<q_rps>"
  Bus Selector/1 -> Bus Creator1/1  "<p_rps>"
  Core/1 -> Bus Selector/1
  Bus Selector/6 -> Bus Creator1/6  "<Az_mpss>"

== system SensLib/ImuSensorModels/Sens_IMU ==
  Core : Inport
  IMU_LocErr : SensLib/ImuSensorModels/IMU_LocErr  VariantControl=VarImu_LocErr
  IMU : Outport
  wires:
  Core/1 -> IMU_LocErr/1
  IMU_LocErr/1 -> IMU/1

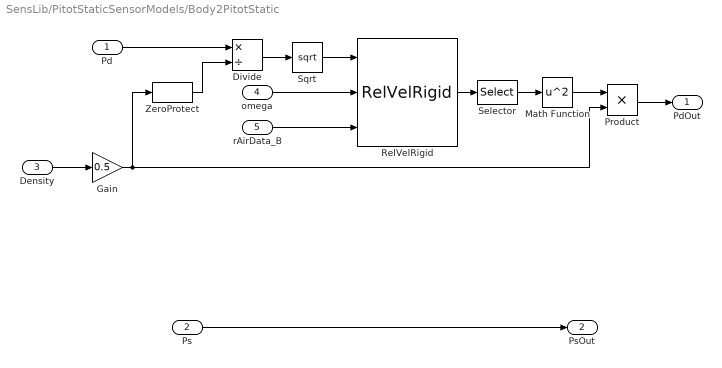
== system SensLib/PitotStaticSensorModels/Body2PitotStatic ==
  Pd : Inport
  Ps : Inport  Port=2
  Density : Inport  Port=3
  omega : Inport  Port=4
  rAirData_B : Inport  Port=5
  Divide : Product  Inputs=*/
  Gain : Gain  Gain=0.5
  Math Function : Math  Operator=square  SaturateOnIntegerOverflow=on
  Product : Product
  RelVelRigid : OpenFlightUtilLib/Kinematics and Dynamics/RelVelRigid
  Selector : Selector  InputPortWidth=3  IndexOptions=Index vector (dialog)  Indices=1  OutputSizes=1
  Sqrt : Sqrt  SaturateOnIntegerOverflow=on
  ZeroProtect : OpenFlightUtilLib/Math/ZeroProtect  epsilon=eps
  PdOut : Outport
  PsOut : Outport  Port=2
  wires:
  ZeroProtect/1 -> Divide/2
  Selector/1 -> Math Function/1
  Math Function/1 -> Product/1
  Gain/1 -> Product/2, ZeroProtect/1
  Density/1 -> Gain/1
  Product/1 -> PdOut/1
  omega/1 -> RelVelRigid/2
  Sqrt/1 -> RelVelRigid/1
  Divide/1 -> Sqrt/1
  Pd/1 -> Divide/1
  RelVelRigid/1 -> Selector/1
  Ps/1 -> PsOut/1
  rAirData_B/1 -> RelVelRigid/3

== system SensLib/PitotStaticSensorModels/Pitot_Err ==
  Core : Inport
  Bus Creator : BusCreator  Inputs=3  OutDataTypeStr=Bus: BusPitot
      settings: AttributesFormatString=%<OutDataTypeStr>  InheritFromInputs=off
  Bus Selector : BusSelector  OutputSignals=AuxVar.qBar_Pa,EnvData.Pressure_kPa,EnvData.Temperature_K
  ErrorModel : SensLib/ErrorModel  enable=sens.errEnable  scf=sens.PdScf  bias=sens.PdBias  sigma=sens.PdSigma  seed=sens.PdSeed  timestep=sens.timeSample_s
  ErrorModel1 : SensLib/ErrorModel  enable=sens.errEnable  scf=sens.PsScf  bias=sens.PsBias  sigma=sens.PsSigma  seed=sens.PsSeed  timestep=sens.timeSample_s
  ErrorModel2 : SensLib/ErrorModel  enable=sens.errEnable  scf=sens.tempScf  bias=sens.tempBias  sigma=sens.tempSigma  seed=sens.tempSeed  timestep=sens.timeSample_s
  Pitot : Outport
  wires:
  Bus Selector/3 -> ErrorModel2/1  "<Temperature_K>"
  Core/1 -> Bus Selector/1
  ErrorModel2/1 -> Bus Creator/3  "temp_K"
  ErrorModel1/1 -> Bus Creator/2  "Ps_Pa"
  ErrorModel/1 -> Bus Creator/1  "Pd_Pa"
  Bus Selector/1 -> ErrorModel/1  "<qBar_Pa>"
  Bus Selector/2 -> ErrorModel1/1  "<Pressure_kPa>"
  Bus Creator/1 -> Pitot/1  "BusPitot"

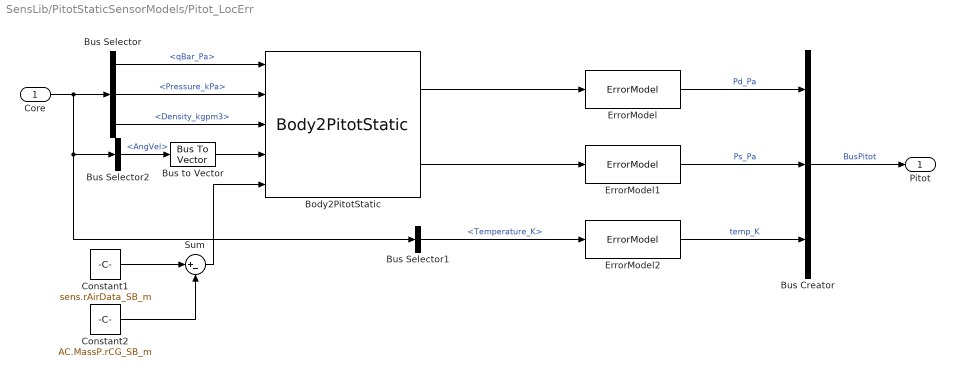
== system SensLib/PitotStaticSensorModels/Pitot_LocErr ==
  Core : Inport
  Body2PitotStatic : SensLib/PitotStaticSensorModels/Body2PitotStatic
  Bus Creator : BusCreator  Inputs=3  OutDataTypeStr=Bus: BusPitot
      settings: AttributesFormatString=%<OutDataTypeStr>  InheritFromInputs=off
  Bus Selector : BusSelector  OutputSignals=AuxVar.qBar_Pa,EnvData.Pressure_kPa,EnvData.Density_kgpm3
  Bus Selector1 : BusSelector  OutputSignals=EnvData.Temperature_K
  Bus Selector2 : BusSelector  OutputSignals=RigidStates.AngVel
  Bus to Vector : BusToVector
  Constant1 : Constant  Value=sens.rAirData_SB_m
      settings: AttributesFormatString=%<Value>
  Constant2 : Constant  Value=AC.MassP.rCG_SB_m
      settings: AttributesFormatString=%<Value>
  ErrorModel : SensLib/ErrorModel  enable=sens.errEnable  scf=sens.PdScf  bias=sens.PdBias  sigma=sens.PdSigma  seed=sens.PdSeed  timestep=sens.timeSample_s
  ErrorModel1 : SensLib/ErrorModel  enable=sens.errEnable  scf=sens.PsScf  bias=sens.PsBias  sigma=sens.PsSigma  seed=sens.PsSeed  timestep=sens.timeSample_s
  ErrorModel2 : SensLib/ErrorModel  enable=sens.errEnable  scf=sens.tempScf  bias=sens.tempBias  sigma=sens.tempSigma  seed=sens.tempSeed  timestep=sens.timeSample_s
  Sum : Sum  Inputs=|+-
  Pitot : Outport
  wires:
  Bus to Vector/1 -> Body2PitotStatic/4
  Bus Selector2/1 -> Bus to Vector/1  "<AngVel>"
  Bus Selector/3 -> Body2PitotStatic/3  "<Density_kgpm3>"
  Bus Selector1/1 -> ErrorModel2/1  "<Temperature_K>"
  ErrorModel/1 -> Bus Creator/1  "Pd_Pa"
  ErrorModel1/1 -> Bus Creator/2  "Ps_Pa"
  ErrorModel2/1 -> Bus Creator/3  "temp_K"
  Core/1 -> Bus Selector1/1, Bus Selector2/1, Bus Selector/1
  Bus Selector/1 -> Body2PitotStatic/1  "<qBar_Pa>"
  Body2PitotStatic/1 -> ErrorModel/1
  Body2PitotStatic/2 -> ErrorModel1/1
  Bus Selector/2 -> Body2PitotStatic/2  "<Pressure_kPa>"
  Constant2/1 -> Sum/2
  Constant1/1 -> Sum/1
  Sum/1 -> Body2PitotStatic/5
  Bus Creator/1 -> Pitot/1  "BusPitot"

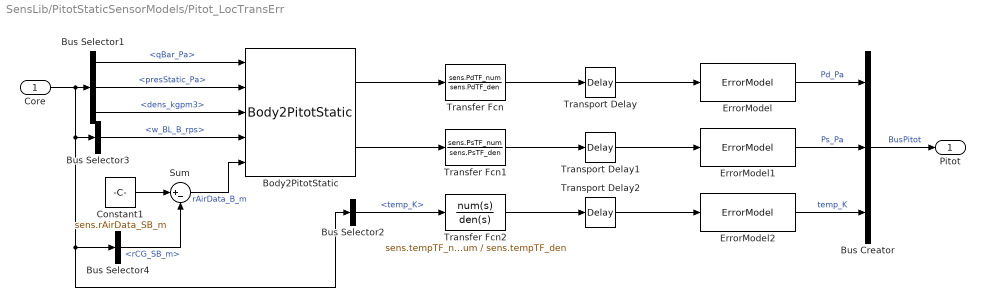
== system SensLib/PitotStaticSensorModels/Pitot_LocTransErr ==
  Core : Inport
  Body2PitotStatic : SensLib/PitotStaticSensorModels/Body2PitotStatic
  Bus Creator : BusCreator  Inputs=3  OutDataTypeStr=Bus: BusPitot
      settings: AttributesFormatString=%<OutDataTypeStr>  InheritFromInputs=off
  Bus Selector1 : BusSelector  OutputSignals=BusAux.BusFlow.qBar_Pa,BusEnv.BusAtmos.presStatic_Pa,BusEnv.BusAtmos.dens_kgpm3
  Bus Selector2 : BusSelector  OutputSignals=BusEnv.BusAtmos.temp_K
  Bus Selector3 : BusSelector  OutputSignals=BusEom.w_BL_B_rps
  Bus Selector4 : BusSelector  OutputSignals=BusEom.rCG_SB_m
  Constant1 : Constant  Value=sens.rAirData_SB_m
      settings: AttributesFormatString=%<Value>
  ErrorModel : SensLib/ErrorModel  enable=sens.errEnable  scf=sens.PdScf  bias=sens.PdBias  sigma=sens.PdSigma  seed=sens.PdSeed  timestep=sens.timeSample_s
  ErrorModel1 : SensLib/ErrorModel  enable=sens.errEnable  scf=sens.PsScf  bias=sens.PsBias  sigma=sens.PsSigma  seed=sens.PsSeed  timestep=sens.timeSample_s
  ErrorModel2 : SensLib/ErrorModel  enable=sens.errEnable  scf=sens.tempScf  bias=sens.tempBias  sigma=sens.tempSigma  seed=sens.tempSeed  timestep=sens.timeSample_s
  Sum : Sum  Inputs=|+-
  Transfer Fcn : TransferFcn  Numerator=sens.PdTF_num  Denominator=sens.PdTF_den
      settings: AttributesFormatString=|
      | %<Numerator>
      | %<Denominator>
  Transfer Fcn1 : TransferFcn  Numerator=sens.PsTF_num  Denominator=sens.PsTF_den
      settings: AttributesFormatString=|
      | %<Numerator>
      | %<Denominator>
  Transfer Fcn2 : TransferFcn  Numerator=sens.tempTF_num  Denominator=sens.tempTF_den
      settings: AttributesFormatString=|
      | %<Numerator>
      | %<Denominator>
  Transport Delay : TransportDelay  DelayTime=sens.PdTimeDelay_s  TransDelayFeedthrough=on  PadeOrder=2
      settings: AttributesFormatString=%<DelayTime>
  Transport Delay1 : TransportDelay  DelayTime=sens.PdTimeDelay_s  TransDelayFeedthrough=on  PadeOrder=2
      settings: AttributesFormatString=%<DelayTime>
  Transport Delay2 : TransportDelay  DelayTime=sens.tempTimeDelay_s  TransDelayFeedthrough=on  PadeOrder=2
      settings: AttributesFormatString=%<DelayTime>
  Pitot : Outport
  wires:
  Bus Creator/1 -> Pitot/1  "BusPitot"
  ErrorModel/1 -> Bus Creator/1  "Pd_Pa"
  ErrorModel1/1 -> Bus Creator/2  "Ps_Pa"
  ErrorModel2/1 -> Bus Creator/3  "temp_K"
  Body2PitotStatic/1 -> Transfer Fcn/1
  Body2PitotStatic/2 -> Transfer Fcn1/1
  Transfer Fcn/1 -> Transport Delay/1
  Transfer Fcn1/1 -> Transport Delay1/1
  Transfer Fcn2/1 -> Transport Delay2/1
  Transport Delay/1 -> ErrorModel/1
  Transport Delay1/1 -> ErrorModel1/1
  Transport Delay2/1 -> ErrorModel2/1
  Bus Selector3/1 -> Body2PitotStatic/4  "<w_BL_B_rps>"
  Bus Selector1/3 -> Body2PitotStatic/3  "<dens_kgpm3>"
  Core/1 -> Bus Selector3/1, Bus Selector4/1, Bus Selector2/1, Bus Selector1/1
  Bus Selector1/1 -> Body2PitotStatic/1  "<qBar_Pa>"
  Bus Selector1/2 -> Body2PitotStatic/2  "<presStatic_Pa>"
  Bus Selector2/1 -> Transfer Fcn2/1  "<temp_K>"
  Bus Selector4/1 -> Sum/2  "<rCG_SB_m>"
  Constant1/1 -> Sum/1
  Sum/1 -> Body2PitotStatic/5  "rAirData_B_m"

== system SensLib/PitotStaticSensorModels/Pitot_Pass ==
  Core : Inport
  Bus Creator : BusCreator  Inputs=3  OutDataTypeStr=Bus: BusPitot
      settings: AttributesFormatString=%<OutDataTypeStr>  InheritFromInputs=off
  Bus Selector : BusSelector  OutputSignals=AuxVar.qBar_Pa,EnvData.Pressure_kPa,EnvData.Temperature_K
  Pitot : Outport
  wires:
  Bus Selector/2 -> Bus Creator/2  "<Pressure_kPa>"
  Bus Selector/1 -> Bus Creator/1  "<qBar_Pa>"
  Bus Creator/1 -> Pitot/1  "BusPitot"
  Core/1 -> Bus Selector/1
  Bus Selector/3 -> Bus Creator/3  "<Temperature_K>"

== system SensLib/PitotStaticSensorModels/Sens_Pitot ==
  Core : Inport
  MassP : Inport  Port=2
  Pitot_Err : SensLib/PitotStaticSensorModels/Pitot_Err  VariantControl=Variant1
  Pitot : Outport
  wires:
  Core/1 -> Pitot_Err/1
  MassP/1 -> Pitot_Err/2
  Pitot_Err/1 -> Pitot/1
